simulink model "mini_project"  (R2024b)
settings: Solver=VariableStepAuto  StartTime=0.0  StopTime=40  FixedStep=0.005  RelTol=1e-3
values from neighbouring files (symbols this model uses):
  g = 9.81    [mini_project_2_par.m]    (also in mini_project_par.m = 9.82)
  Ic = diag([ 2 ; 2 ; 4 ])    [mini_project_2_par.m]
  m = 4    [mini_project_2_par.m]    (also in mini_project_par.m = 0.725)
  M_RB = [ m*eye(3) , zeros(3) ; zeros(3) , Ic ]    [mini_project_2_par.m]
libraries: slpidlib x3, simulink_extras x2, aerolibutil x2, vrlib x1, simulink x1
settings Model: VariantFading=off  Creator=peter  LastModifiedBy=ander

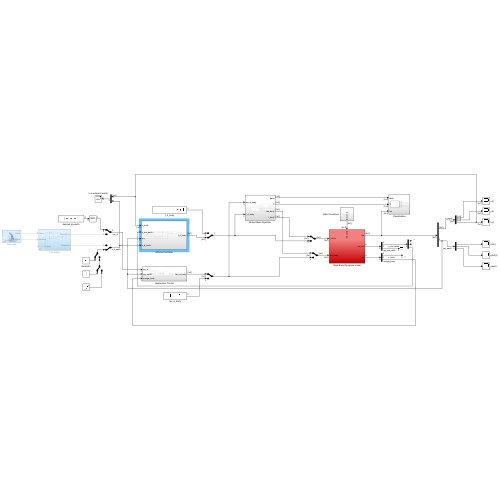
[thumbnail: Simulink's stored preview of the top-level diagram]
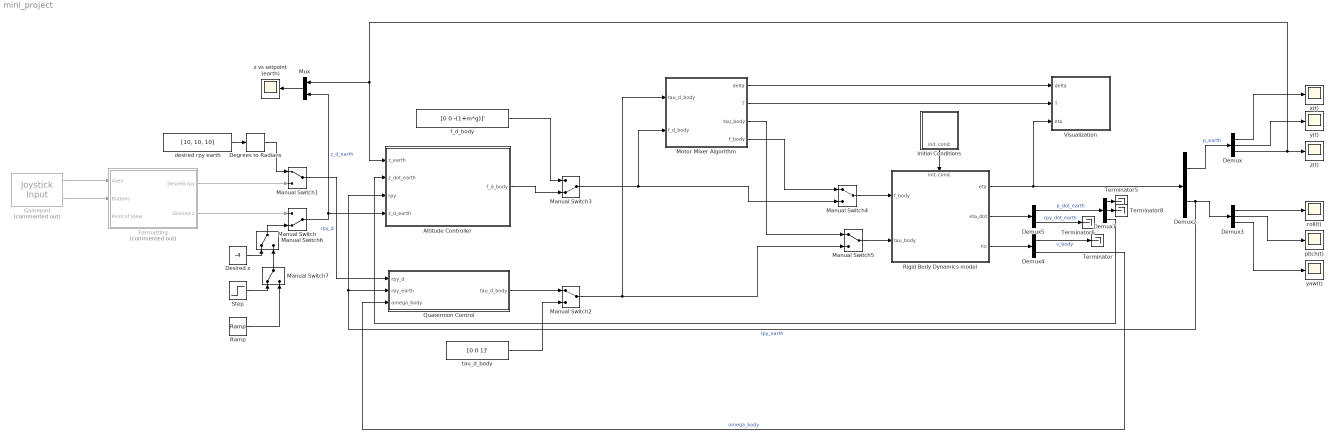
== system mini_project ==
  Altitude Controller : Subsystem
  Degrees to Radians : simulink_extras/Transformations/Degrees to Radians
  Demux : Demux  Outputs=3
  Demux2 : Demux  Outputs=2
  Demux3 : Demux  Outputs=3
  Demux4 : Demux  Outputs=2
  Demux5 : Demux  Outputs=2
  Demux7 : Demux  Outputs=3
  Desired z : Constant  Value=-4
  Formatting : Subsystem  Commented=on
  Gamepad : vrlib/Joystick Input  Commented=on  joyid=1  adjustports=on  forcefeed=off
  Initial Conditions : Subsystem
  Manual Switch : ManualSwitch  CurrentSetting=0
  Manual Switch{1..2,4..7} (6 alike) : ManualSwitch
  Manual Switch3 : ManualSwitch  CurrentSetting=0
  Motor Mixer Algorithm : Subsystem
  Mux : Mux  Inputs=2
  Quaternion Control : Subsystem
  Ramp : simulink/Sources/Ramp  slope=-2  start=1  InitialOutput=0
  Rigid Body Dynamics model : Subsystem
      settings: PortSchema="{\"entries\":[{\"content\":{\"sides\":[{\"content\":{\"connectorIds\":[\"In1\",\"In2\"]},\"type\":\"ConnectorPlacement.EquallySpacedRectSide\",\"uuid\":\"c5c2dfb8-9ff8-4aa4-96a6-7fa0d886c51f\"},{\"content\":{\"connectorIds\":[\"Out1\",\"Out2\",\"Out3\"],\"side\":\"RIGHT\"},\"type\":\"ConnectorPlacement.EquallySpacedRectSide\",\"uuid\":\"2d7c7d5c-4ac5-4ebd-b09f-6a78733e851d\"},{\"content\":{\"connectorIds\":[\"In3\"],\"side\":\"TOP\"},\"type\":\"ConnectorPlacement.EquallySpacedRectSide\",\"uuid\":\"cf3a786d-06ed-46d4-985b-5c210afb13ec\"}]},\"type\":\"ConnectorPlacement.EquallySpacedConnector\",\"uuid\":\"cd57f0e6-7b9c-4392-8478-6e8af8e2560e\"}],\"packageUris\":[\"http://schema.mathworks.com/mf0/Connector/R2020b\"],\"version\":\"1.0\"}"
  Step : Step  After=-2  SampleTime=0
  Terminator{,5..6,8} (4 alike) : Terminator
  Visualization : Subsystem
  desired rpy earth : Constant  Value=[10, 10, 10]
  f_d_body : Constant  Value=[0 0 -(1+m*g)]'
  pitch(t) : Scope
  roll(t) : Scope
  tau_d_body : Constant  Value=[0 0 1]'
  x(t) : Scope
  y(t) : Scope
  yaw(t) : Scope
  z vs setpoint (earth) : Scope
  z(t) : Scope
  wires:
  Rigid Body Dynamics model/1(eta) -> Demux2/1, Visualization/3(eta)
  f_d_body/1 -> Manual Switch3/1
  Manual Switch3/1 -> Manual Switch4/2, Motor Mixer Algorithm/2(f_d_body)
  Rigid Body Dynamics model/3(nu) -> Demux4/1
  Demux4/1 -> Terminator/1  "v_body"
  Demux2/1 -> Demux/1  "p_earth"
  Demux5/1 -> Demux7/1  "p_dot_earth"
  Demux5/2 -> Terminator6/1  "rpy_dot_earth"
  Rigid Body Dynamics model/2(eta_dot) -> Demux5/1
  Demux7/1 -> Terminator5/1
  Demux7/2 -> Terminator8/1
  Gamepad/2 -> Formatting/2(Buttons)
  Gamepad/1 -> Formatting/1(Axes)
  Formatting/1(Desired rpy) -> Manual Switch1/2
  Formatting/2(Desired z) -> Manual Switch/1
  Manual Switch1/1 -> Quaternion Control/1(rpy_d)  "rpy_d"
  desired rpy earth/1 -> Degrees to Radians/1
  Manual Switch4/1 -> Rigid Body Dynamics model/1(f_body)
  Manual Switch5/1 -> Rigid Body Dynamics model/2(tau_body)
  Manual Switch2/1 -> Motor Mixer Algorithm/1(tau_d_body), Manual Switch5/2
  Demux4/2 -> Quaternion Control/3(omega_body)  "omega_body"
  Demux7/3 -> Altitude Controller/2(z_dot_earth)
  Manual Switch/1 -> Mux/2, Altitude Controller/4(z_d_earth)  "z_d_earth"
  Altitude Controller/1(f_d_body) -> Manual Switch3/2
  Motor Mixer Algorithm/3(tau_body) -> Manual Switch5/1
  Motor Mixer Algorithm/4(f_body) -> Manual Switch4/1
  Motor Mixer Algorithm/2(T) -> Visualization/2(T)
  Motor Mixer Algorithm/1(delta) -> Visualization/1(delta)
  Quaternion Control/1(tau_d_body) -> Manual Switch2/1
  tau_d_body/1 -> Manual Switch2/2
  Initial Conditions/1(init. cond.) -> Rigid Body Dynamics model/3(init. cond.)
  Demux2/2 -> Quaternion Control/2(rpy_earth), Altitude Controller/3(rpy), Demux3/1  "rpy_earth"
  Demux/3 -> z(t)/1, Altitude Controller/1(z_earth), Mux/1
  Demux/1 -> x(t)/1
  Demux/2 -> y(t)/1
  Demux3/1 -> roll(t)/1
  Demux3/2 -> pitch(t)/1
  Demux3/3 -> yaw(t)/1
  Mux/1 -> z vs setpoint (earth)/1
  Manual Switch6/1 -> Manual Switch/2
  Desired z/1 -> Manual Switch6/1
  Step/1 -> Manual Switch7/1
  Ramp/1 -> Manual Switch7/2
  Manual Switch7/1 -> Manual Switch6/2
  Degrees to Radians/1 -> Manual Switch1/1

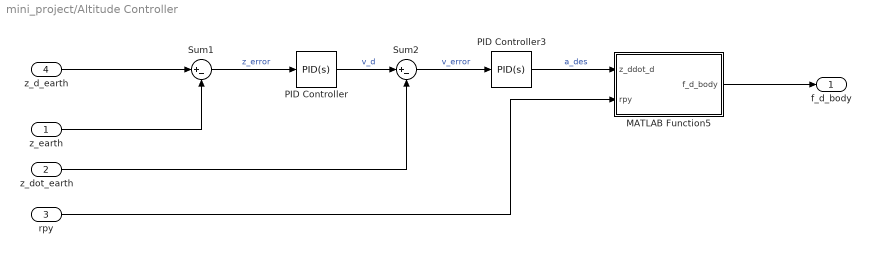
== system mini_project/Altitude Controller ==
  z_earth : Inport
  z_dot_earth : Inport  Port=2
  rpy : Inport  Port=3
  z_d_earth : Inport  Port=4
  MATLAB Function5 : MATLAB Function  TreatAsAtomicUnit=on
  PID Controller : slpidlib/PID Controller  Controller=PID  Form=Parallel  TimeDomain=Continuous-time  UseExternalTs=off  SampleTime=-1  IntegratorMethod=Forward Euler  FilterMethod=Forward Euler  ControllerParametersSource=internal  P=15  I=8  UseKiTs=off  D=1  UseExternalDerivativeSource=off  N=100  UseFilter=on  TunerSelectOption=Transfer Function Based (PID Tuner App)  InitialConditionSource=internal  InitialConditionForIntegrator=0  InitialConditionForFilter=0  DifferentiatorICPrevScaledInput=0  ExternalReset=none  TrackingMode=off  Kt=1  LimitOutput=off  SatLimitsSource=internal  UpperSaturationLimit=inf  LowerSaturationLimit=-inf  LinearizeAsGain=on  AntiWindupMode=none  Kb=1  LimitIntegrator=off  UpperIntegratorSaturationLimit=inf  LowerIntegratorSaturationLimit=-inf  POutMin=[]  POutMax=[]  IOutMin=[]  IOutMax=[]  DOutMin=[]  DOutMax=[]  NOutMin=[]  NOutMax=[]  SumOutMin=[]  SumOutMax=[]  SaturationOutMin=[]  SaturationOutMax=[]  PParamMin=[]  PParamMax=[]  IParamMin=[]  IParamMax=[]  DParamMin=[]  DParamMax=[]  NParamMin=[]  NParamMax=[]  KbParamMin=[]  KbParamMax=[]  KtParamMin=[]  KtParamMax=[]  KbOutMin=[]  KbOutMax=[]  KtOutMin=[]  KtOutMax=[]  IntegratorOutMin=[]  IntegratorOutMax=[]  FilterOutMin=[]  FilterOutMax=[]  SumI1OutMin=[]  SumI1OutMax=[]  SumI2OutMin=[]  SumI2OutMax=[]  SumI3OutMin=[]  SumI3OutMax=[]  SumI4OutMin=[]  SumI4OutMax=[]  SumDOutMin=[]  SumDOutMax=[]  DifferentiatorOutMin=[]  DifferentiatorOutMax=[]  FilterDiffOutCoefMin=[]  FilterDiffOutCoefMax=[]  ReciprocalOutMin=[]  ReciprocalOutMax=[]  SumDenOutMin=[]  SumDenOutMax=[]  SumNumOutMin=[]  SumNumOutMax=[]  DivideOutMin=[]  DivideOutMax=[]  UdiffTsProdOutMin=[]  UdiffTsProdOutMax=[]  NTsProdOutMin=[]  NTsProdOutMax=[]  UintegralTsProdOutMin=[]  UintegralTsProdOutMax=[]  UngainTsProdOutMin=[]  UngainTsProdOutMax=[]  ClampingZeroOutDataTypeStr=Inherit: Inherit via back propagation  ClampingZeroOutMin=[]  ClampingZeroOutMax=[]  FilterDenConstantOutDataTypeStr=Inherit: Inherit via back propagation  FilterDenConstantOutMin=[]  FilterDenConstantOutMax=[]  PCopyOutDataTypeStr=Inherit: Inherit via back propagation  PCopyOutMin=[]  PCopyOutMax=[]  NCopyOutDataTypeStr=Inherit: Inherit via back propagation  NCopyOutMin=[]  NCopyOutMax=[]  IntegratorContinuousStateAttributes=''  IntegratorStateMustResolveToSignalObject=off  IntegratorRTWStateStorageClass=Auto  FilterContinuousStateAttributes=''  FilterStateMustResolveToSignalObject=off  FilterRTWStateStorageClass=Auto  ParallelPVariant=InternalParameters  IdealPVariant=Disabled  IVariant=InternalParameters  DVariant=InternalParameters  IntegratorVariant=Continuous  SatVariant=Disabled  AWVariant=Passthrough  PCopyVariant=Disabled  TRVariant=Disabled  FdbkBlocksVariant=Forward  IdealPFdbkVariant=Disabled  SatFdbkVariant=Disabled  DerivativeFilterVariant=ContFilter  NVariant=InternalParameters  NCopyVariant=Disabled  FilterICVariant=InternalICsFilter  IntegratorICVariant=InternalICs  ExternalResetVariant=Disabled  TRSumVariant=Passthrough  SumFdbkVariant=Disabled  SumVariant=Sum_PID  TsampFilterVariant=InternalTs  TsampNgainVariant=Passthrough  TsampIntegralVariant=Disabled_SignalSpec  ExternalSaturationOutDataTypeStr=Inherit: Same as second input  DerivativeSourceVariant=ErrorSignal  PreIntVariant=InternalPreInt
  PID Controller3 : slpidlib/PID Controller  Controller=PID  Form=Parallel  TimeDomain=Continuous-time  UseExternalTs=off  SampleTime=-1  IntegratorMethod=Forward Euler  FilterMethod=Forward Euler  ControllerParametersSource=internal  P=1  I=0  UseKiTs=off  D=0  UseExternalDerivativeSource=off  N=100  UseFilter=on  TunerSelectOption=Transfer Function Based (PID Tuner App)  InitialConditionSource=internal  InitialConditionForIntegrator=0  InitialConditionForFilter=0  DifferentiatorICPrevScaledInput=0  ExternalReset=none  TrackingMode=off  Kt=1  LimitOutput=off  SatLimitsSource=internal  UpperSaturationLimit=inf  LowerSaturationLimit=-inf  LinearizeAsGain=on  AntiWindupMode=none  Kb=1  LimitIntegrator=off  UpperIntegratorSaturationLimit=inf  LowerIntegratorSaturationLimit=-inf  POutMin=[]  POutMax=[]  IOutMin=[]  IOutMax=[]  DOutMin=[]  DOutMax=[]  NOutMin=[]  NOutMax=[]  SumOutMin=[]  SumOutMax=[]  SaturationOutMin=[]  SaturationOutMax=[]  PParamMin=[]  PParamMax=[]  IParamMin=[]  IParamMax=[]  DParamMin=[]  DParamMax=[]  NParamMin=[]  NParamMax=[]  KbParamMin=[]  KbParamMax=[]  KtParamMin=[]  KtParamMax=[]  KbOutMin=[]  KbOutMax=[]  KtOutMin=[]  KtOutMax=[]  IntegratorOutMin=[]  IntegratorOutMax=[]  FilterOutMin=[]  FilterOutMax=[]  SumI1OutMin=[]  SumI1OutMax=[]  SumI2OutMin=[]  SumI2OutMax=[]  SumI3OutMin=[]  SumI3OutMax=[]  SumI4OutMin=[]  SumI4OutMax=[]  SumDOutMin=[]  SumDOutMax=[]  DifferentiatorOutMin=[]  DifferentiatorOutMax=[]  FilterDiffOutCoefMin=[]  FilterDiffOutCoefMax=[]  ReciprocalOutMin=[]  ReciprocalOutMax=[]  SumDenOutMin=[]  SumDenOutMax=[]  SumNumOutMin=[]  SumNumOutMax=[]  DivideOutMin=[]  DivideOutMax=[]  UdiffTsProdOutMin=[]  UdiffTsProdOutMax=[]  NTsProdOutMin=[]  NTsProdOutMax=[]  UintegralTsProdOutMin=[]  UintegralTsProdOutMax=[]  UngainTsProdOutMin=[]  UngainTsProdOutMax=[]  ClampingZeroOutDataTypeStr=Inherit: Inherit via back propagation  ClampingZeroOutMin=[]  ClampingZeroOutMax=[]  FilterDenConstantOutDataTypeStr=Inherit: Inherit via back propagation  FilterDenConstantOutMin=[]  FilterDenConstantOutMax=[]  PCopyOutDataTypeStr=Inherit: Inherit via back propagation  PCopyOutMin=[]  PCopyOutMax=[]  NCopyOutDataTypeStr=Inherit: Inherit via back propagation  NCopyOutMin=[]  NCopyOutMax=[]  IntegratorContinuousStateAttributes=''  IntegratorStateMustResolveToSignalObject=off  IntegratorRTWStateStorageClass=Auto  FilterContinuousStateAttributes=''  FilterStateMustResolveToSignalObject=off  FilterRTWStateStorageClass=Auto  ParallelPVariant=InternalParameters  IdealPVariant=Disabled  IVariant=InternalParameters  DVariant=InternalParameters  IntegratorVariant=Continuous  SatVariant=Disabled  AWVariant=Passthrough  PCopyVariant=Disabled  TRVariant=Disabled  FdbkBlocksVariant=Forward  IdealPFdbkVariant=Disabled  SatFdbkVariant=Disabled  DerivativeFilterVariant=ContFilter  NVariant=InternalParameters  NCopyVariant=Disabled  FilterICVariant=InternalICsFilter  IntegratorICVariant=InternalICs  ExternalResetVariant=Disabled  TRSumVariant=Passthrough  SumFdbkVariant=Disabled  SumVariant=Sum_PID  TsampFilterVariant=InternalTs  TsampNgainVariant=Passthrough  TsampIntegralVariant=Disabled_SignalSpec  ExternalSaturationOutDataTypeStr=Inherit: Same as second input  DerivativeSourceVariant=ErrorSignal  PreIntVariant=InternalPreInt
  Sum1 : Sum  Inputs=|+-
  Sum2 : Sum  Inputs=|+-
  f_d_body : Outport
  wires:
  PID Controller/1 -> Sum2/1  "v_d"
  Sum2/1 -> PID Controller3/1  "v_error"
  Sum1/1 -> PID Controller/1  "z_error"
  MATLAB Function5/1(f_d_body) -> f_d_body/1
  rpy/1 -> MATLAB Function5/2(rpy)
  z_d_earth/1 -> Sum1/1
  PID Controller3/1 -> MATLAB Function5/1(z_ddot_d)  "a_des"
  z_earth/1 -> Sum1/2
  z_dot_earth/1 -> Sum2/2

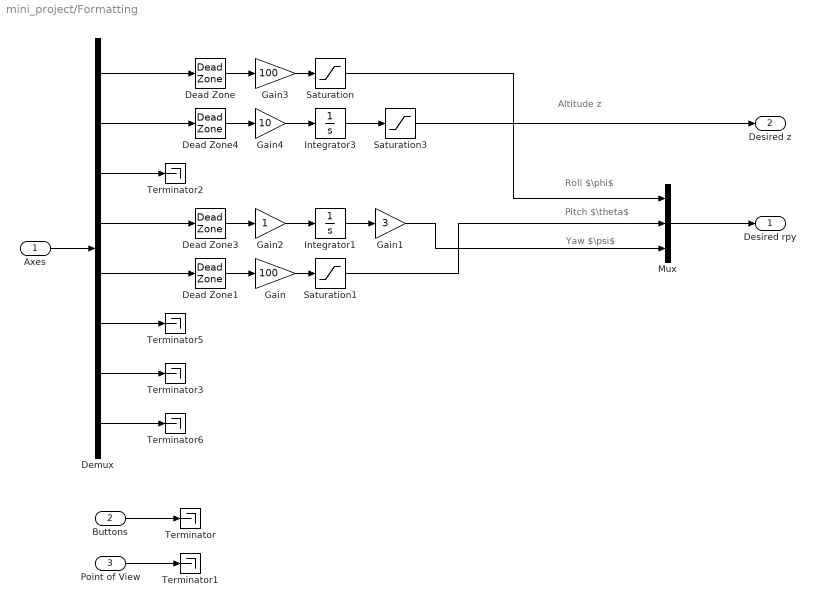
== system mini_project/Formatting ==
  note: Roll $\phi$
  note: Pitch $\theta$
  note: Yaw $\psi$
  note: Altitude z
  Axes : Inport
  Buttons : Inport  Port=2
  Point of View : Inport  Port=3
  Dead Zone{,1,3..4} (4 alike) : DeadZone  LowerValue=-0.2  UpperValue=0.2
  Demux : Demux  Outputs=8
  Gain : Gain  Gain=100
  Gain1 : Gain  Gain=3
  Gain2 : Gain
  Gain3 : Gain  Gain=100
  Gain4 : Gain  Gain=10
  Integrator1 : Integrator
  Integrator3 : Integrator  InitialCondition=-2
  Mux : Mux  Inputs=3
  Saturation : Saturate  UpperLimit=pi/4  LowerLimit=-pi/4
  Saturation1 : Saturate  UpperLimit=pi/4  LowerLimit=-pi/4
  Saturation3 : Saturate  UpperLimit=0  LowerLimit=-100
  Terminator{,1..3,5..6} (6 alike) : Terminator
  Desired rpy : Outport
  Desired z : Outport  Port=2
  wires:
  Buttons/1 -> Terminator/1
  Axes/1 -> Demux/1
  Demux/6 -> Terminator5/1
  Dead Zone1/1 -> Gain/1
  Dead Zone/1 -> Gain3/1
  Dead Zone3/1 -> Gain2/1
  Point of View/1 -> Terminator1/1
  Mux/1 -> Desired rpy/1
  Demux/1 -> Dead Zone/1
  Gain4/1 -> Integrator3/1
  Dead Zone4/1 -> Gain4/1
  Demux/2 -> Dead Zone4/1
  Integrator3/1 -> Saturation3/1
  Demux/7 -> Terminator3/1
  Gain2/1 -> Integrator1/1
  Gain/1 -> Saturation1/1
  Gain3/1 -> Saturation/1
  Saturation/1 -> Mux/1
  Saturation1/1 -> Mux/2
  Gain1/1 -> Mux/3
  Integrator1/1 -> Gain1/1
  Saturation3/1 -> Desired z/1
  Demux/8 -> Terminator6/1
  Demux/4 -> Dead Zone3/1
  Demux/5 -> Dead Zone1/1
  Demux/3 -> Terminator2/1

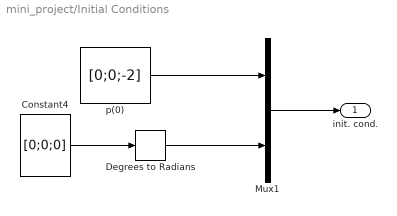
== system mini_project/Initial Conditions ==
  Constant4 : Constant  Value=[0;0;0]  VectorParams1D=off
  Degrees to Radians : simulink_extras/Transformations/Degrees to Radians
  Mux1 : Mux  Inputs=2
  p(0) : Constant  Value=[0;0;-2]  VectorParams1D=off
  init. cond. : Outport
  wires:
  Degrees to Radians/1 -> Mux1/2
  p(0)/1 -> Mux1/1
  Mux1/1 -> init. cond./1
  Constant4/1 -> Degrees to Radians/1

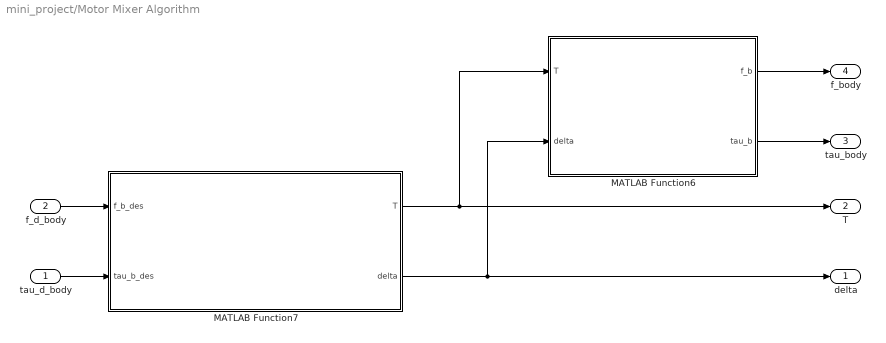
== system mini_project/Motor Mixer Algorithm ==
  tau_d_body : Inport
  f_d_body : Inport  Port=2
  MATLAB Function6 : MATLAB Function  TreatAsAtomicUnit=on
  MATLAB Function7 : MATLAB Function  TreatAsAtomicUnit=on
  delta : Outport
  T : Outport  Port=2
  tau_body : Outport  Port=3
  f_body : Outport  Port=4
  wires:
  MATLAB Function7/1(T) -> MATLAB Function6/1(T), T/1
  MATLAB Function7/2(delta) -> MATLAB Function6/2(delta), delta/1
  MATLAB Function6/1(f_b) -> f_body/1
  MATLAB Function6/2(tau_b) -> tau_body/1
  f_d_body/1 -> MATLAB Function7/1(f_b_des)
  tau_d_body/1 -> MATLAB Function7/2(tau_b_des)

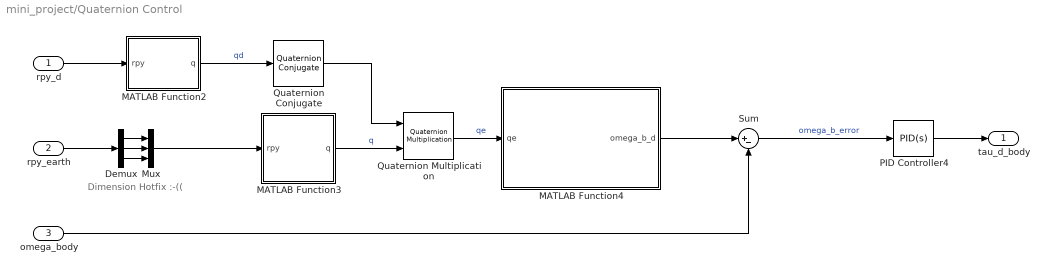
== system mini_project/Quaternion Control ==
  note: Dimension Hotfix :-((
  rpy_d : Inport
  rpy_earth : Inport  Port=2
  omega_body : Inport  Port=3
  Demux : Demux  Outputs=3
  MATLAB Function2 : MATLAB Function  TreatAsAtomicUnit=on
  MATLAB Function3 : MATLAB Function  TreatAsAtomicUnit=on
  MATLAB Function4 : MATLAB Function  TreatAsAtomicUnit=on
  Mux : Mux  Inputs=3
  PID Controller4 : slpidlib/PID Controller  Controller=PID  Form=Parallel  TimeDomain=Continuous-time  UseExternalTs=off  SampleTime=-1  IntegratorMethod=Forward Euler  FilterMethod=Forward Euler  ControllerParametersSource=internal  P=[25, 25, 25]  I=[0.1, 0.1, 0.1]  UseKiTs=off  D=[1,1, 1]  UseExternalDerivativeSource=off  N=100  UseFilter=on  TunerSelectOption=Transfer Function Based (PID Tuner App)  InitialConditionSource=internal  InitialConditionForIntegrator=0  InitialConditionForFilter=0  DifferentiatorICPrevScaledInput=0  ExternalReset=none  TrackingMode=off  Kt=1  LimitOutput=off  SatLimitsSource=internal  UpperSaturationLimit=inf  LowerSaturationLimit=-inf  LinearizeAsGain=on  AntiWindupMode=none  Kb=1  LimitIntegrator=off  UpperIntegratorSaturationLimit=inf  LowerIntegratorSaturationLimit=-inf  POutMin=[]  POutMax=[]  IOutMin=[]  IOutMax=[]  DOutMin=[]  DOutMax=[]  NOutMin=[]  NOutMax=[]  SumOutMin=[]  SumOutMax=[]  SaturationOutMin=[]  SaturationOutMax=[]  PParamMin=[]  PParamMax=[]  IParamMin=[]  IParamMax=[]  DParamMin=[]  DParamMax=[]  NParamMin=[]  NParamMax=[]  KbParamMin=[]  KbParamMax=[]  KtParamMin=[]  KtParamMax=[]  KbOutMin=[]  KbOutMax=[]  KtOutMin=[]  KtOutMax=[]  IntegratorOutMin=[]  IntegratorOutMax=[]  FilterOutMin=[]  FilterOutMax=[]  SumI1OutMin=[]  SumI1OutMax=[]  SumI2OutMin=[]  SumI2OutMax=[]  SumI3OutMin=[]  SumI3OutMax=[]  SumI4OutMin=[]  SumI4OutMax=[]  SumDOutMin=[]  SumDOutMax=[]  DifferentiatorOutMin=[]  DifferentiatorOutMax=[]  FilterDiffOutCoefMin=[]  FilterDiffOutCoefMax=[]  ReciprocalOutMin=[]  ReciprocalOutMax=[]  SumDenOutMin=[]  SumDenOutMax=[]  SumNumOutMin=[]  SumNumOutMax=[]  DivideOutMin=[]  DivideOutMax=[]  UdiffTsProdOutMin=[]  UdiffTsProdOutMax=[]  NTsProdOutMin=[]  NTsProdOutMax=[]  UintegralTsProdOutMin=[]  UintegralTsProdOutMax=[]  UngainTsProdOutMin=[]  UngainTsProdOutMax=[]  ClampingZeroOutDataTypeStr=Inherit: Inherit via back propagation  ClampingZeroOutMin=[]  ClampingZeroOutMax=[]  FilterDenConstantOutDataTypeStr=Inherit: Inherit via back propagation  FilterDenConstantOutMin=[]  FilterDenConstantOutMax=[]  PCopyOutDataTypeStr=Inherit: Inherit via back propagation  PCopyOutMin=[]  PCopyOutMax=[]  NCopyOutDataTypeStr=Inherit: Inherit via back propagation  NCopyOutMin=[]  NCopyOutMax=[]  IntegratorContinuousStateAttributes=''  IntegratorStateMustResolveToSignalObject=off  IntegratorRTWStateStorageClass=Auto  FilterContinuousStateAttributes=''  FilterStateMustResolveToSignalObject=off  FilterRTWStateStorageClass=Auto  ParallelPVariant=InternalParameters  IdealPVariant=Disabled  IVariant=InternalParameters  DVariant=InternalParameters  IntegratorVariant=Continuous  SatVariant=Disabled  AWVariant=Passthrough  PCopyVariant=Disabled  TRVariant=Disabled  FdbkBlocksVariant=Forward  IdealPFdbkVariant=Disabled  SatFdbkVariant=Disabled  DerivativeFilterVariant=ContFilter  NVariant=InternalParameters  NCopyVariant=Disabled  FilterICVariant=InternalICsFilter  IntegratorICVariant=InternalICs  ExternalResetVariant=Disabled  TRSumVariant=Passthrough  SumFdbkVariant=Disabled  SumVariant=Sum_PID  TsampFilterVariant=InternalTs  TsampNgainVariant=Passthrough  TsampIntegralVariant=Disabled_SignalSpec  ExternalSaturationOutDataTypeStr=Inherit: Same as second input  DerivativeSourceVariant=ErrorSignal  PreIntVariant=InternalPreInt
  Quaternion Conjugate : aerolibutil/Quaternion Conjugate
  Quaternion Multiplication : aerolibutil/Quaternion Multiplication
  Sum : Sum  Inputs=|+-
  tau_d_body : Outport
  wires:
  Sum/1 -> PID Controller4/1  "omega_b_error"
  MATLAB Function2/1(q) -> Quaternion Conjugate/1  "qd"
  Quaternion Conjugate/1 -> Quaternion Multiplication/1
  Quaternion Multiplication/1 -> MATLAB Function4/1(qe)  "qe"
  MATLAB Function3/1(q) -> Quaternion Multiplication/2  "q"
  PID Controller4/1 -> tau_d_body/1
  rpy_d/1 -> MATLAB Function2/1(rpy)
  MATLAB Function4/1(omega_b_d) -> Sum/1
  omega_body/1 -> Sum/2
  Demux/1 -> Mux/1
  Demux/2 -> Mux/2
  Demux/3 -> Mux/3
  rpy_earth/1 -> Demux/1
  Mux/1 -> MATLAB Function3/1(rpy)

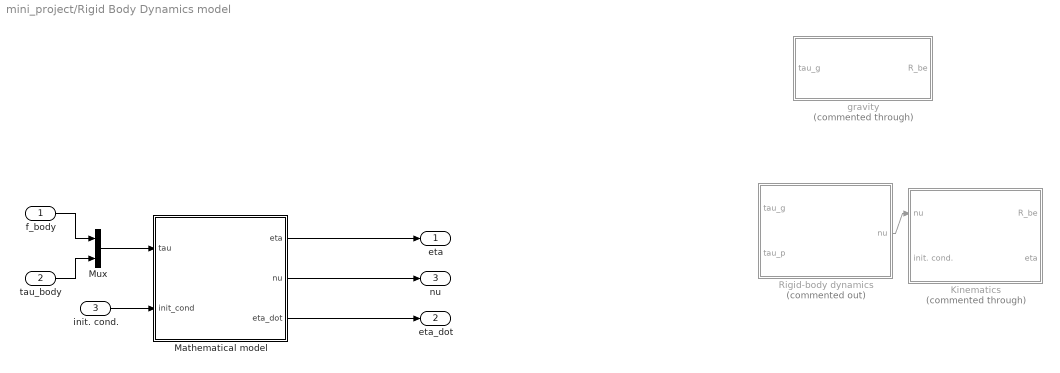
== system mini_project/Rigid Body Dynamics model ==
  f_body : Inport
  tau_body : Inport  Port=2
  init. cond. : Inport  Port=3
  Kinematics : Subsystem  Commented=through
  Mathematical model : Subsystem
  Mux : Mux  Inputs=2
  Rigid-body dynamics : Subsystem  Commented=on
  gravity : Subsystem  Commented=through
  eta : Outport
  eta_dot : Outport  Port=2
  nu : Outport  Port=3
  wires:
  Rigid-body dynamics/1(nu) -> Kinematics/1(nu)
  tau_body/1 -> Mux/2
  f_body/1 -> Mux/1
  Mux/1 -> Mathematical model/1(tau)
  init. cond./1 -> Mathematical model/2(init_cond)
  Mathematical model/2(nu) -> nu/1
  Mathematical model/1(eta) -> eta/1
  Mathematical model/3(eta_dot) -> eta_dot/1

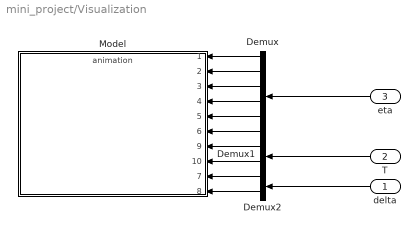
== system mini_project/Visualization ==
  delta : Inport
  T : Inport  Port=2
  eta : Inport  Port=3
  Demux : Demux  Outputs=6
  Demux1 : Demux  Outputs=2
  Demux2 : Demux  Outputs=2
  Model : ModelReference  ModelNameDialog=animation.slx  SimulationMode=Normal  ModelReferenceVersion=1.15
      settings: PortSchema="{\"entries\":[{\"content\":{\"sides\":[{\"content\":{\"connectorIds\":[\"In1\",\"In2\",\"In3\",\"In4\",\"In5\",\"In6\",\"In9\",\"In10\",\"In7\",\"In8\"]},\"type\":\"ConnectorPlacement.EquallySpacedRectSide\",\"uuid\":\"93ed0a95-d791-4fc8-9088-15197577fe2b\"},{\"content\":{\"side\":\"RIGHT\"},\"type\":\"ConnectorPlacement.EquallySpacedRectSide\",\"uuid\":\"345d8874-0f4a-47e1-9f54-67e066b67754\"},{\"content\":{\"side\":\"TOP\"},\"type\":\"ConnectorPlacement.EquallySpacedRectSide\",\"uuid\":\"f55a885d-5fd3-4d0d-a64b-a37e54015f91\"}]},\"type\":\"ConnectorPlacement.EquallySpacedConnector\",\"uuid\":\"7215b92f-3597-4c90-a055-6ed313f77b19\"}],\"packageUris\":[\"http://schema.mathworks.com/mf0/Connector/R2020b\"],\"version\":\"1.0\"}"
  wires:
  Demux1/2 -> Model/10
  Demux2/2 -> Model/8
  Demux1/1 -> Model/9
  Demux/3 -> Model/3
  Demux/4 -> Model/4
  Demux/2 -> Model/2
  Demux/5 -> Model/5
  eta/1 -> Demux/1
  Demux2/1 -> Model/7
  Demux/6 -> Model/6
  Demux/1 -> Model/1
  delta/1 -> Demux2/1
  T/1 -> Demux1/1

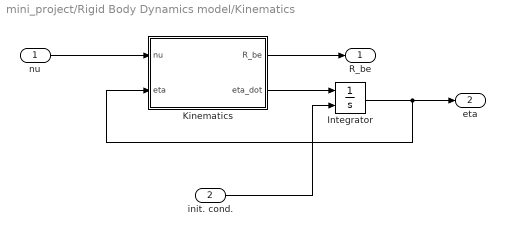
== system mini_project/Rigid Body Dynamics model/Kinematics ==
  nu : Inport
  init. cond. : Inport  Port=2
  Integrator : Integrator  InitialConditionSource=external  InitialCondition=[0;0;-10;0;pi/2;0]
  Kinematics : MATLAB Function  TreatAsAtomicUnit=on
  R_be : Outport
  eta : Outport  Port=2
  wires:
  Kinematics/1(R_be) -> R_be/1
  Kinematics/2(eta_dot) -> Integrator/1
  nu/1 -> Kinematics/1(nu)
  init. cond./1 -> Integrator/2
  Integrator/1 -> eta/1, Kinematics/2(eta)

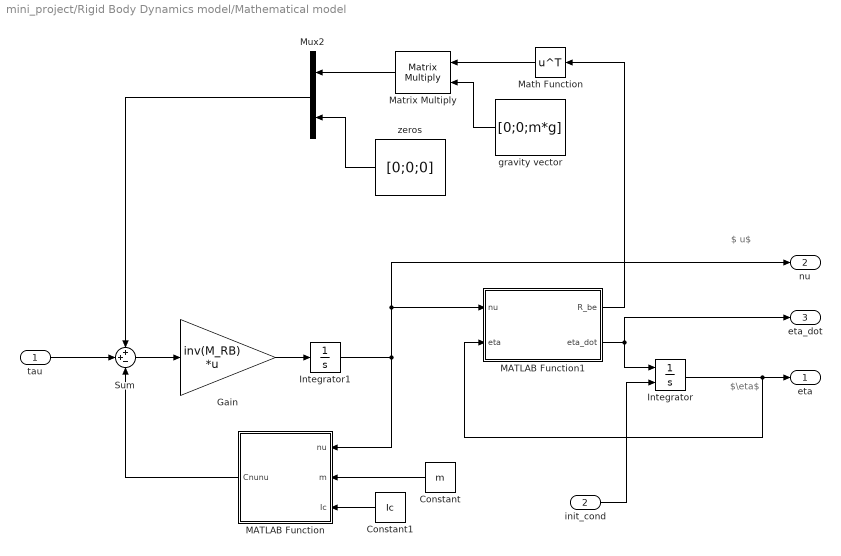
== system mini_project/Rigid Body Dynamics model/Mathematical model ==
  note: $\eta$
  note: $\nu$
  tau : Inport
  init_cond : Inport  Port=2
  Constant : Constant  Value=m
  Constant1 : Constant  Value=Ic  VectorParams1D=off
  Gain : Gain  Gain=inv(M_RB)  Multiplication=Matrix(K*u) (u vector)
  Integrator : Integrator  InitialConditionSource=external  InitialCondition=[0;0;-10;0;pi/2;0]
  Integrator1 : Integrator  InitialCondition=[0;0;0;0;0;0]
  MATLAB Function : MATLAB Function  TreatAsAtomicUnit=on
  MATLAB Function1 : MATLAB Function  TreatAsAtomicUnit=on
  Math Function : Math  Operator=transpose
  Matrix Multiply : Product  Multiplication=Matrix(*)
  Mux2 : Mux  Inputs=2
  Sum : Sum  Inputs=++-
  gravity vector : Constant  Value=[0;0;m*g]  VectorParams1D=off
  zeros : Constant  Value=[0;0;0]  VectorParams1D=off
  eta : Outport
  nu : Outport  Port=2
  eta_dot : Outport  Port=3
  wires:
  Integrator/1 -> eta/1, MATLAB Function1/2(eta)
  Integrator1/1 -> MATLAB Function1/1(nu), nu/1, MATLAB Function/1(nu)
  MATLAB Function1/2(eta_dot) -> Integrator/1, eta_dot/1
  Constant/1 -> MATLAB Function/2(m)
  Constant1/1 -> MATLAB Function/3(Ic)
  Gain/1 -> Integrator1/1
  Sum/1 -> Gain/1
  init_cond/1 -> Integrator/2
  gravity vector/1 -> Matrix Multiply/2
  Matrix Multiply/1 -> Mux2/1
  zeros/1 -> Mux2/2
  Math Function/1 -> Matrix Multiply/1
  MATLAB Function1/1(R_be) -> Math Function/1
  tau/1 -> Sum/2
  MATLAB Function/1(Cnunu) -> Sum/3
  Mux2/1 -> Sum/1

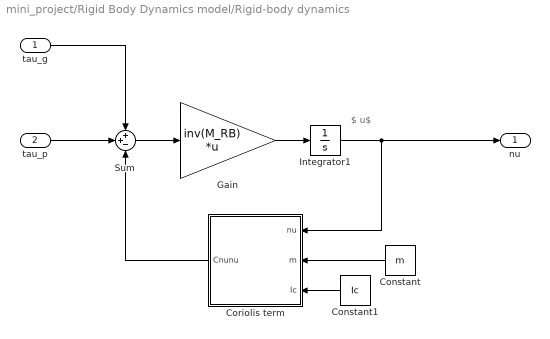
== system mini_project/Rigid Body Dynamics model/Rigid-body dynamics ==
  note: $\nu$
  tau_g : Inport
  tau_p : Inport  Port=2
  Constant : Constant  Value=m
  Constant1 : Constant  Value=Ic  VectorParams1D=off
  Coriolis term : MATLAB Function  TreatAsAtomicUnit=on
  Gain : Gain  Gain=inv(M_RB)  Multiplication=Matrix(K*u) (u vector)
  Integrator1 : Integrator  InitialCondition=[0;0;0;0;0;0]
  Sum : Sum  Inputs=++-
  nu : Outport
  wires:
  Integrator1/1 -> nu/1, Coriolis term/1(nu)
  Constant/1 -> Coriolis term/2(m)
  Sum/1 -> Gain/1
  tau_p/1 -> Sum/2
  Coriolis term/1(Cnunu) -> Sum/3
  Constant1/1 -> Coriolis term/3(Ic)
  Gain/1 -> Integrator1/1
  tau_g/1 -> Sum/1

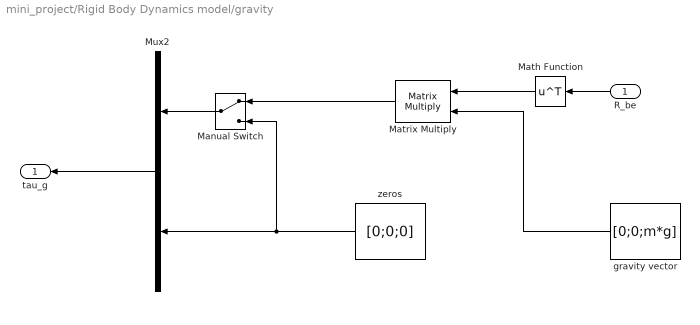
== system mini_project/Rigid Body Dynamics model/gravity ==
  R_be : Inport
  Manual Switch : ManualSwitch
  Math Function : Math  Operator=transpose
  Matrix Multiply : Product  Multiplication=Matrix(*)
  Mux2 : Mux  Inputs=2
  gravity vector : Constant  Value=[0;0;m*g]  VectorParams1D=off
  zeros : Constant  Value=[0;0;0]  VectorParams1D=off
  tau_g : Outport
  wires:
  Matrix Multiply/1 -> Manual Switch/1
  Manual Switch/1 -> Mux2/1
  Mux2/1 -> tau_g/1
  gravity vector/1 -> Matrix Multiply/2
  zeros/1 -> Mux2/2, Manual Switch/2
  Math Function/1 -> Matrix Multiply/1
  R_be/1 -> Math Function/1

== matlab function mini_project/Motor Mixer Algorithm/MATLAB Function6 ==
  data: f_b output; tau_b output; T input; delta input
function [f_b, tau_b] = compute_body_forces(T, delta)

    T1 = T(1);
    T2 = T(2);
    delta1 = delta(1);
    delta2 = delta(2);

    L = 0.5;  % half-length between motors (along x-axis)
    D = 0.2;  % vertical offset from CoM to rotor plane

    % Thrust vector components in y and z (z points down)
    F1_y = T1 * sin(delta1);
    F1_z = T1 * cos(delta1);

    F2_y = T2 * sin(delta2);
    F2_z = T2 * cos(delta2);

    % Net body forces (no x force because tilting is only in y-z)
    Fx = 0;
    Fy = F1_y + F2_y;
    Fz = F1_z + F2_z;

    % Body torques:
    Tau_x = D * (F1_y + F2_y);            % Rolling moment due to lateral forces and height D
    Tau_y = L * (F1_z - F2_z);            % Pitching moment due to thrust difference
    Tau_z = L * (F1_y - F2_y);            % Yawing moment due to lateral force difference

    f_b = [Fx, Fy, Fz]';
    tau_b = [Tau_x, Tau_y, Tau_z]';
end

== matlab function mini_project/Rigid Body Dynamics model/Kinematics/Kinematics ==
  data: R_be output; nu input; eta input; eta_dot output
function [R_be,eta_dot] = J_Theta(nu,eta)

% Euler angle extraction
phi = eta(4);
theta = eta(5);
psi = eta(6);

R_xphi = [ 1 0 0 ; 0 cos(phi) -sin(phi) ; 0 sin(phi) cos(phi) ];
R_ytheta = [ cos(theta) 0 sin(theta) ; 0 1 0 ; -sin(theta) 0 cos(theta) ];
R_zpsi = [ cos(psi) -sin(psi) 0 ; sin(psi) cos(psi) 0 ; 0 0 1 ];

% rotation matrix
R_be = R_zpsi * R_ytheta * R_xphi;

% angular velocity transformation
T_Theta = [ 1 sin(phi)*tan(theta) cos(phi)*tan(theta) ; 0 cos(phi) -sin(phi) ; 0 sin(phi)/cos(theta) cos(phi)/cos(theta) ];

J_Theta = [ R_be , zeros(3) ; zeros(3) , T_Theta ];

eta_dot = J_Theta*nu;

== matlab function mini_project/Motor Mixer Algorithm/MATLAB Function7 ==
  settings: updateMethod=DISCRETE
  data: f_b_des input; tau_b_des input; T output; delta output
function [T, delta] = get_motor_thrusts_and_angles(f_b_des, tau_b_des)

f_b_z_des = f_b_des(3);
tau_b_x_des = tau_b_des(1);
tau_b_y_des = tau_b_des(2);
tau_b_z_des = tau_b_des(3);

% Run external script solve_bicopter.m to solve the optimization problem
[T1, T2, delta1, delta2] = solve_bicopter(f_b_z_des, tau_b_x_des, tau_b_y_des, tau_b_z_des);
   
% Return motor thrusts and servo angles
T = [T1, T2];
delta = [delta1, delta2];
end

== matlab function mini_project/Rigid Body Dynamics model/Rigid-body dynamics/Coriolis term ==
  data: nu input; Cnunu output; m input; Ic input
function Cnunu = fcn(nu,m,Ic)

v = nu(1:3);  % linear velocities (expressed in the body frame)
omega = nu(4:6); % angular velocities (expressed in the body frame)


Cnunu = [ cross(omega,m*v) ; -cross(Ic*omega,omega) ];

== matlab function mini_project/Quaternion Control/MATLAB Function2 ==
  data: rpy input; q output
function q = euler2quat(rpy) %eul has to be [yaw pitch roll]
    roll = rpy(1);
    pitch = rpy(2);
    yaw_unwrapped = rpy(3);
    yaw = mod(yaw_unwrapped + pi, 2*pi) - pi;
    
    eul = [yaw; pitch; roll];
    q = eul2quat(eul', "ZYX");
end

== matlab function mini_project/Quaternion Control/MATLAB Function3 ==
  data: rpy input; q output
function q = euler2quat(rpy) %eul has to be [yaw pitch roll]
    roll = rpy(1);
    pitch = rpy(2);
    yaw_unwrapped = rpy(3);
    yaw = mod(yaw_unwrapped + pi, 2*pi) - pi;

    eul = [yaw; pitch; roll];
    q = eul2quat(eul', "ZYX");
end

== matlab function mini_project/Quaternion Control/MATLAB Function4 ==
  data: qe input; omega_b_d output
function omega_b_d = get_desired_angular_velocity(qe)
    nue = qe(1);
    ee = qe(2:4);

    ee = reshape(ee, 1, 3); 
    
    phi = 2 * atan2(norm(ee), nue);
    omega_b_d = zeros(1, 3);
     
    % Avoid division by zero if phi is very small
    if abs(sin(phi / 2)) > 1e-6
        omega_b_d = -1 * sign(nue) * (phi / sin(phi / 2)) * ee;
    end
end

== matlab function mini_project/Altitude Controller/MATLAB Function5 ==
  data: z_ddot_d input; f_d_body output; rpy input
function f_d_body = get_force(z_ddot_d, rpy)
    m = 4; % kg
    g = 9.82; % m/s^2

    % Wrap angles to valid range
    roll_wrapped = mod(rpy(1) + pi, 2*pi) - pi;
    pitch_wrapped = mod(rpy(2) + pi, 2*pi) - pi;
    yaw_wrapped = mod(rpy(3) + pi, 2*pi) - pi;
    rpy_wrapped = [yaw_wrapped, pitch_wrapped, roll_wrapped];

    rotmZYX = eul2rotm(rpy_wrapped, 'ZYX');  % Assumes [yaw, pitch, roll]

    f_g = [0; 0; m * g];
    a_d = [0; 0; z_ddot_d];

    % Total desired force in earth fixed frame (+ clamping)
    f_d_earth = m * a_d - f_g;
    if f_d_earth(3) > 0
        f_d_earth(3) = 0;
    end
    f_d_body = inv(rotmZYX) * f_d_earth;
end

== matlab function mini_project/Rigid Body Dynamics model/Mathematical model/MATLAB Function ==
  data: nu input; Cnunu output; m input; Ic input
function Cnunu = fcn(nu,m,Ic)

v = nu(1:3);  % linear velocities (expressed in the body frame)
omega = nu(4:6); % angular velocities (expressed in the body frame)


Cnunu = [ cross(omega,m*v) ; -cross(Ic*omega,omega) ];

== matlab function mini_project/Rigid Body Dynamics model/Mathematical model/MATLAB Function1 ==
  data: R_be output; nu input; eta input; eta_dot output
function [R_be,eta_dot] = J_Theta(nu,eta)

% Euler angle extraction
phi = eta(4);
theta = eta(5);
psi = eta(6);

R_xphi = [ 1 0 0 ; 0 cos(phi) -sin(phi) ; 0 sin(phi) cos(phi) ];
R_ytheta = [ cos(theta) 0 sin(theta) ; 0 1 0 ; -sin(theta) 0 cos(theta) ];
R_zpsi = [ cos(psi) -sin(psi) 0 ; sin(psi) cos(psi) 0 ; 0 0 1 ];

% rotation matrix
R_be = R_zpsi * R_ytheta * R_xphi;

% angular velocity transformation
T_Theta = [ 1 sin(phi)*tan(theta) cos(phi)*tan(theta) ; 0 cos(phi) -sin(phi) ; 0 sin(phi)/cos(theta) cos(phi)/cos(theta) ];

J_Theta = [ R_be , zeros(3) ; zeros(3) , T_Theta ];

eta_dot = J_Theta*nu;
